simulink model "LBR_MED_Simul"  (R2026a)
settings: Solver=VariableStepAuto
libraries: LBR_MED_Lib x1
settings Model: Creator=ivovilamowski  LastModifiedBy=ivovilamowski

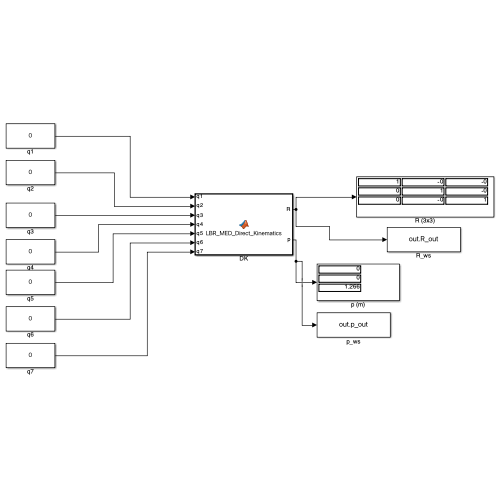
[thumbnail: Simulink's stored preview of the top-level diagram]
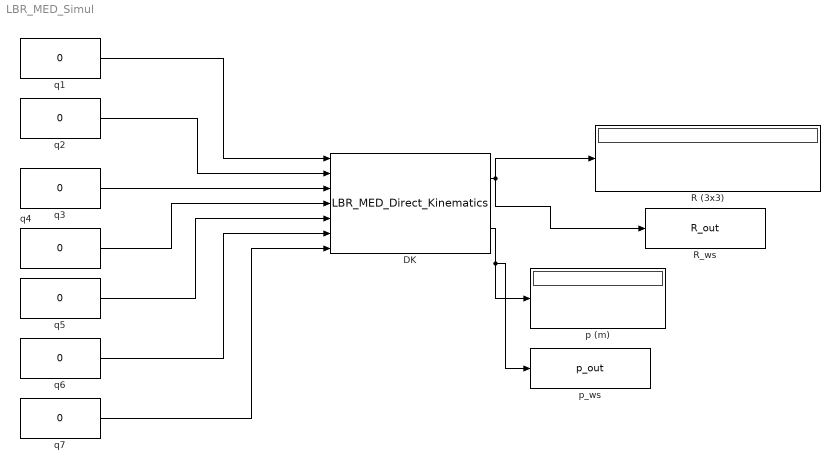
== system LBR_MED_Simul ==
  DK : LBR_MED_Lib/LBR_MED_Direct_Kinematics  SystemSampleTime=-1  VariantActivationTime=update diagram  EmptyChoice=off  PassThrough=off  PassThroughVariantControl=(default)  EmptyChoiceVariantControl=(default)  AllowFlexibleInterface=on  Latency=0  AutoFrameSizeCalculation=off
  R (3x3) : Display
  R_ws : ToWorkspace  VariableName=R_out  SaveFormat=Timeseries  SampleTime=-1
  p (m) : Display
  p_ws : ToWorkspace  VariableName=p_out  SaveFormat=Timeseries  SampleTime=-1
  q{1..7} (7 alike) : Constant  Value=0
  wires:
  q1/1 -> DK/1
  q2/1 -> DK/2
  q3/1 -> DK/3
  q4/1 -> DK/4
  q5/1 -> DK/5
  q6/1 -> DK/6
  q7/1 -> DK/7
  DK/1 -> R_ws/1, R (3x3)/1
  DK/2 -> p (m)/1, p_ws/1
